simulink model "AS"  (R2021b)
settings: Solver=VariableStepAuto  StartTime=0.0  StopTime=10.0  RelTol=1e-3
values from neighbouring files (symbols this model uses):
  alpha = (1 + sqrt(1 - 4*Td/Ti))/2    [avaliaAS.m]    (also in compararAntiWindUps.m)
  antiwindupON = 0    [avaliaAS.m]    (also in compararAntiWindUps.m = 1)
  controlador = projetarControlador(planta)    [avaliaAS.m]    (also in avaliaBC1.m; avaliaBC2.m = projetarControladorPI(planta); avaliaCI.m; avaliaMalhaPura.m)
  planta = obterPlanta()    [avaliaAS.m]    (also in avaliaBC1.m; avaliaBC2.m; avaliaCI.m; avaliaMalhaPura.m)
  Td = controlador.Kd/controlador.Kp    [avaliaAS.m]    (also in compararAntiWindUps.m; projetarControlador.m = Kd/Kp; projetarControladorPI.m = Kd/Kp)
  Ti = controlador.Kp/controlador.Ki    [avaliaAS.m]    (also in compararAntiWindUps.m; projetarControlador.m = Kp/Ki; projetarControladorPI.m = Kp/Ki)
settings Model: Creator=gagan  LastModifiedBy=emanu
settings SolverCC: ZeroCrossAlgorithm=Adaptive
settings DebuggingCC: IgnoredZcDiagnostic=none

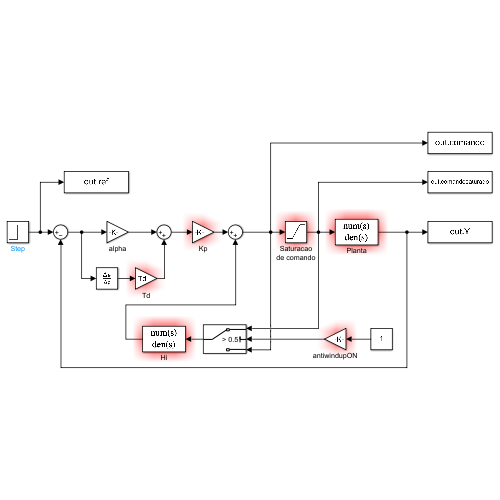
[thumbnail: Simulink's stored preview of the top-level diagram]
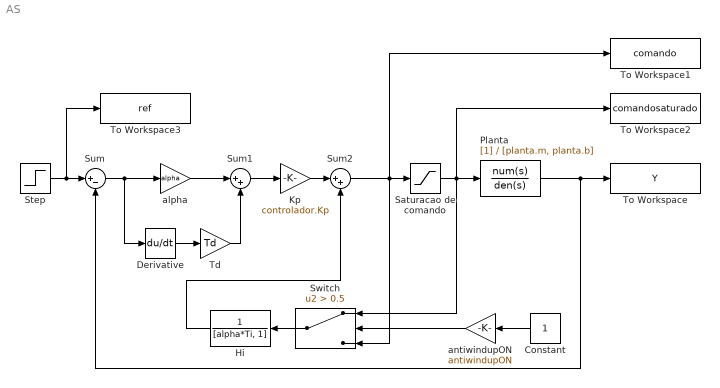
== system AS ==
  Constant : Constant
  Derivative : Derivative
  Hi : TransferFcn  Denominator=[alpha*Ti, 1]  ParameterTunability=Optimized
  Kp : Gain  Gain=controlador.Kp
  Planta : TransferFcn  Denominator=[planta.m, planta.b]  ParameterTunability=Optimized
  Saturacao de comando : Saturate  UpperLimit=planta.comandoNominal  LowerLimit=-planta.comandoNominal
  Step : Step  SampleTime=0
  Sum : Sum  Inputs=|+-
  Sum1 : Sum  Inputs=|++
  Sum2 : Sum  Inputs=|++
  Switch : Switch  Criteria=u2 > Threshold  Threshold=0.5
  Td : Gain  Gain=Td
  To Workspace : ToWorkspace  VariableName=Y  SaveFormat=Structure With Time  SampleTime=-1
  To Workspace1 : ToWorkspace  VariableName=comando  SaveFormat=Structure With Time  SampleTime=-1
  To Workspace2 : ToWorkspace  VariableName=comandosaturado  SaveFormat=Structure With Time  SampleTime=-1
  To Workspace3 : ToWorkspace  VariableName=ref  SaveFormat=Structure With Time  SampleTime=-1
  alpha : Gain  Gain=alpha
  antiwindupON : Gain  Gain=antiwindupON
  wires:
  Sum2/1 -> To Workspace1/1, Switch/3, Saturacao de comando/1
  Planta/1 -> To Workspace/1, Sum/2
  Step/1 -> To Workspace3/1, Sum/1
  Kp/1 -> Sum2/1
  Saturacao de comando/1 -> Planta/1, To Workspace2/1, Switch/1
  Hi/1 -> Sum2/2
  alpha/1 -> Sum1/1
  Sum/1 -> alpha/1, Derivative/1
  Derivative/1 -> Td/1
  Td/1 -> Sum1/2
  Switch/1 -> Hi/1
  antiwindupON/1 -> Switch/2
  Constant/1 -> antiwindupON/1
  Sum1/1 -> Kp/1
